simulink model "symlab"  (R2021b)
settings: Solver=VariableStepAuto  StartTime=0.0  StopTime=czas_symulacji  MaxStep=0.01  RelTol=1e-3
undefined symbols (not defined in the file): Cvp, Cvw, dTzad, dTzew, K, Kcp, Kcw, Kcwp, Ki, Kp, qg0, t0, t0x, Tp, Tp0, Twew0, Tzad, Tzew0
settings Model: Creator=Ovocsiak  LastModifiedBy=Ovocsiak
settings DataIOCC: ReturnWorkspaceOutputs=off

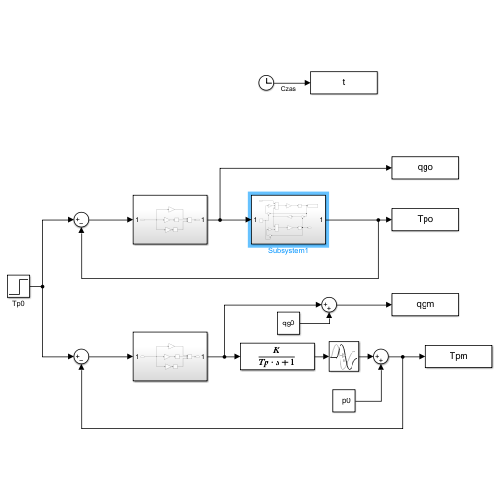
[thumbnail: Simulink's stored preview of the top-level diagram]
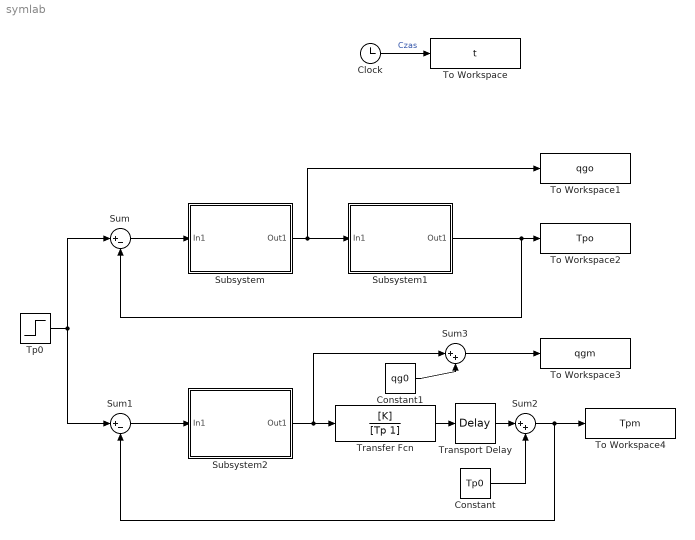
== system symlab ==
  Clock : Clock
  Constant : Constant  Value=Tp0
  Constant1 : Constant  Value=qg0
  Subsystem : Subsystem
  Subsystem1 : Subsystem
  Subsystem2 : Subsystem
  Sum : Sum  Inputs=|+-
  Sum1 : Sum  Inputs=|+-
  Sum2 : Sum  Inputs=|++
  Sum3 : Sum  Inputs=|++
  To Workspace : ToWorkspace  VariableName=t  SampleTime=-1
  To Workspace1 : ToWorkspace  VariableName=qgo  SampleTime=-1
  To Workspace2 : ToWorkspace  VariableName=Tpo  SampleTime=-1
  To Workspace3 : ToWorkspace  VariableName=qgm  SampleTime=-1
  To Workspace4 : ToWorkspace  VariableName=Tpm  SampleTime=-1
  Tp0 : Step  Time=t0  Before=Tzad  After=Tzad + dTzad  SampleTime=0
  Transfer Fcn : TransferFcn  Numerator=[K]  Denominator=[Tp 1]
  Transport Delay : TransportDelay  DelayTime=t0x
  wires:
  Clock/1 -> To Workspace/1  "Czas"
  Sum/1 -> Subsystem/1(In1)
  Subsystem/1(Out1) -> Subsystem1/1(In1), To Workspace1/1
  Subsystem1/1(Out1) -> Sum/2, To Workspace2/1
  Subsystem2/1(Out1) -> Sum3/1, Transfer Fcn/1
  Sum1/1 -> Subsystem2/1(In1)
  Tp0/1 -> Sum/1, Sum1/1
  Transfer Fcn/1 -> Transport Delay/1
  Transport Delay/1 -> Sum2/1
  Sum2/1 -> Sum1/2, To Workspace4/1
  Constant/1 -> Sum2/2
  Sum3/1 -> To Workspace3/1
  Constant1/1 -> Sum3/2

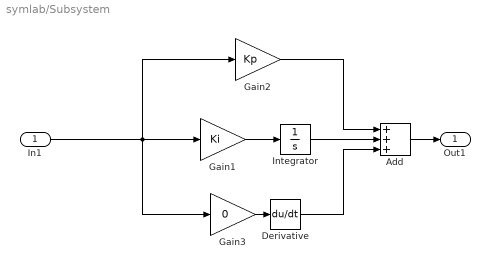
== system symlab/Subsystem ==
  In1 : Inport
  Add : Sum  Inputs=+++
  Derivative : Derivative
  Gain1 : Gain  Gain=Ki
  Gain2 : Gain  Gain=Kp
  Gain3 : Gain  Gain=0
  Integrator : Integrator  InitialCondition=qg0
  Out1 : Outport
  wires:
  Gain2/1 -> Add/1
  Derivative/1 -> Add/3
  Add/1 -> Out1/1
  Integrator/1 -> Add/2
  In1/1 -> Gain3/1, Gain1/1, Gain2/1
  Gain1/1 -> Integrator/1
  Gain3/1 -> Derivative/1

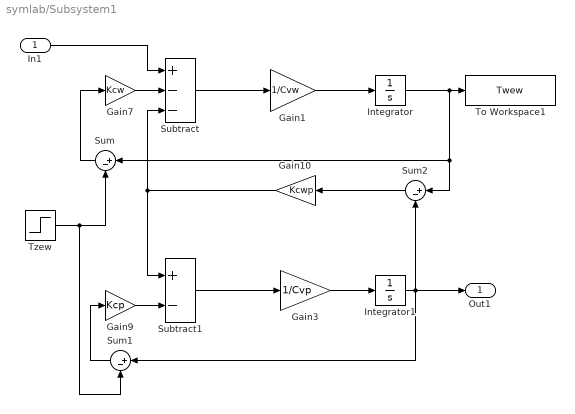
== system symlab/Subsystem1 ==
  In1 : Inport
  Gain1 : Gain  Gain=1/Cvw
  Gain10 : Gain  Gain=Kcwp
  Gain3 : Gain  Gain=1/Cvp
  Gain7 : Gain  Gain=Kcw
  Gain9 : Gain  Gain=Kcp
  Integrator : Integrator  InitialCondition=Twew0
  Integrator1 : Integrator  InitialCondition=Tp0
  Subtract : Sum  Inputs=+--
  Subtract1 : Sum  Inputs=+-
  Sum : Sum  Inputs=|+-
  Sum1 : Sum  Inputs=|+-
  Sum2 : Sum  Inputs=|+-
  To Workspace1 : ToWorkspace  VariableName=Twew  SampleTime=-1
  Tzew : Step  Time=t0  Before=Tzew0  After=Tzew0 + dTzew  SampleTime=0
  Out1 : Outport
  wires:
  Gain9/1 -> Subtract1/2
  Gain10/1 -> Subtract1/1, Subtract/3
  Sum1/1 -> Gain9/1
  Subtract/1 -> Gain1/1
  Gain1/1 -> Integrator/1
  Subtract1/1 -> Gain3/1
  Gain7/1 -> Subtract/2
  Integrator/1 -> Sum/1, Sum2/1, To Workspace1/1
  Sum/1 -> Gain7/1
  Tzew/1 -> Sum/2, Sum1/2
  Integrator1/1 -> Out1/1, Sum1/1, Sum2/2
  Gain3/1 -> Integrator1/1
  Sum2/1 -> Gain10/1
  In1/1 -> Subtract/1

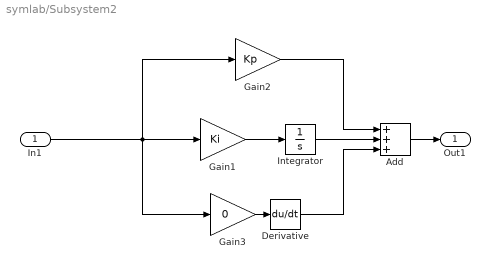
== system symlab/Subsystem2 ==
  In1 : Inport
  Add : Sum  Inputs=+++
  Derivative : Derivative
  Gain1 : Gain  Gain=Ki
  Gain2 : Gain  Gain=Kp
  Gain3 : Gain  Gain=0
  Integrator : Integrator
  Out1 : Outport
  wires:
  Gain3/1 -> Derivative/1
  Gain1/1 -> Integrator/1
  In1/1 -> Gain2/1, Gain1/1, Gain3/1
  Integrator/1 -> Add/2
  Add/1 -> Out1/1
  Derivative/1 -> Add/3
  Gain2/1 -> Add/1
